simulink model "LEGO_SW"  (R2023a)
settings: Solver=VariableStepAuto  StartTime=0.0  StopTime=45  RelTol=1e-3  EnableMultiTasking=on
values from neighbouring files (symbols this model uses):
  A1 = [0,0,1,0 ... (first row only)    [run_LEGO_SW.m]
  A2 = [0,1;0,-W^2/(2*R^2)*(Kfrac+b+b_bar)/Denom]    [run_LEGO_SW.m]
  B1 = [0;0;2*(M*R*L+M*L^2+Jpsi)*Kt/Rdc/q;-2*((2*m+M)*R^2+2*J+M*R*L)*Kt/Rdc/q]    [run_LEGO_SW.m]
  B2 = [0;-W/R*Kt/Rdc/Denom]    [run_LEGO_SW.m]
  C1 = [1,0,0,0;0,0,0,1]    [run_LEGO_SW.m]
  C2 = [1,0]    [run_LEGO_SW.m]
  D1 = [0;0]    [run_LEGO_SW.m]
  D2 = 0    [run_LEGO_SW.m]
  KDtheta = -1    [run_LEGO_SW.m]
  KIpsi = -100    [run_LEGO_SW.m]
  KItheta = w_0^2*KDtheta    (= -0.8464)    [run_LEGO_SW.m]
  Kopenloop = -A2(2,2)/B2(2,1)    [run_LEGO_SW.m]
  KPphi = 6    [run_LEGO_SW.m]
  KPpsi = -10    [run_LEGO_SW.m]
  KPtheta = KDtheta * 2 * w_0 * zeta    (= -0.92)    [run_LEGO_SW.m]
  R = 0.027    [run_LEGO_SW.m]
undefined symbols (not defined in the file or in its folder): sigbuilder_block
libraries: slpidlib x2
settings Model: Creator=KostasM  LastModifiedBy=Lab5
settings SolverCC: AlgebraicLoopSolver=TrustRegion
settings DataIOCC: LimitDataPoints=on  ReturnWorkspaceOutputs=off
settings OptimizationCC: LifeSpan=inf
settings DebuggingCC: UnconnectedInputMsg=warning  UnconnectedOutputMsg=warning  UnconnectedLineMsg=warning  AllowSymbolicDim=off  SFUnexpectedBacktrackingDiag=warning  SFNoUnconditionalDefaultTransitionDiag=warning  SFExecutionAtInitializationDiag=none  ArithmeticOperatorsInVariantConditions=warning
settings ModelReferenceCC: EnableRefExpFcnMdlSchedulingChecks=on  PropagateSignalLabelsOutOfModel=off
settings SFSimCC: SimUseLocalCustomCode=off  CustomCodeUndefinedFunction=UseInterfaceOnly
settings RTWCC: RTWUseLocalCustomCode=off  DLArmComputeVersion=19.05
settings CodeAppCC: StateflowObjectComments=on
settings GRTTargetCC: TargetLangStandard=C89/C90 (ANSI)
settings ConfigComp: CovMetricSettings=dw  CovSaveCumulativeToWorkspaceVar=on  CovSaveSingleToWorkspaceVar=on  CovExternalEMLEnable=off

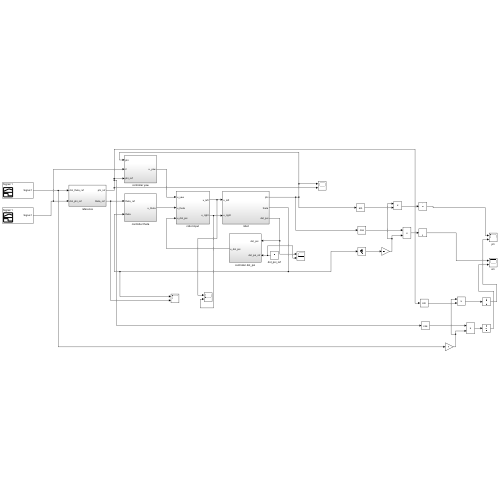
[thumbnail: Simulink's stored preview of the top-level diagram]
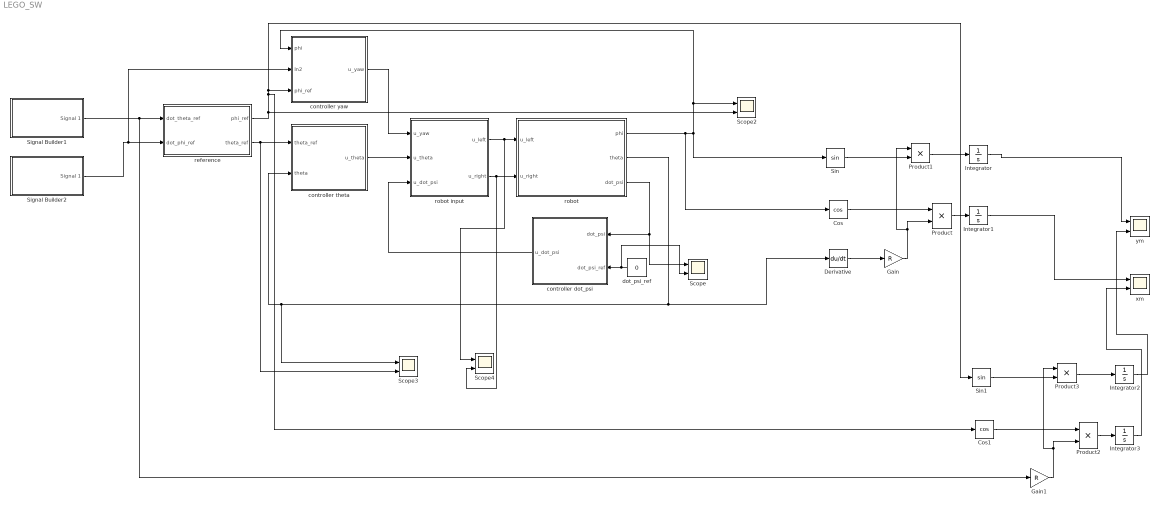
== system LEGO_SW ==
  Cos : Trigonometry  Operator=cos
  Cos1 : Trigonometry  Operator=cos
  Derivative : Derivative
  Gain : Gain  Gain=R
  Gain1 : Gain  Gain=R
  Integrator{,1..3} (4 alike) : Integrator
  Product{,1..3} (4 alike) : Product
  Scope{,2..4} (4 alike) : Scope  NumInputPorts=2
  Signal Builder1 : Subsystem  Tag=STV Subsys  LoadFcn=sigbuilder_block('load');  StartFcn=sigbuilder_block('start');  StopFcn=sigbuilder_block('stop');  ClipboardFcn=sigbuilder_block('clipboard');  mask(Sigbuilder block){tuvar=[0:10]}
      mask help: Sigbuilder GUI
      mask init:
      | if ~strcmp(get_param(bdroot(gcbh),'SimulationStatus'),'stopped') tuvar = sigbuilder_block('maskInit'); end
      settings: CopyFcn=sigbuilder_block('copy');  DeleteFcn=sigbuilder_block('delete');  ModelCloseFcn=sigbuilder_block('modelClose');  PreSaveFcn=sigbuilder_block('preSave');  PauseFcn=sigbuilder_block('pause')  ContinueFcn=sigbuilder_block('continue')  NameChangeFcn=sigbuilder_block('namechange');  OpenFcn=sigbuilder_block('open',[181.5 38.5 516 349.5 ]);  CloseFcn=sigbuilder_block('close');
      mask Display: plot(0, 0, 100, 100,[2, 2, 32, 32, 2], [68, 8, 8, 68, 68],[32, 2], [38, 38], [32, 19, 2],[53, 60, 44], [32, 17, 17, 2],[16, 16, 31, 31]);txt = getActiveGroup(gcbh);text(2, 100, txt,'verticalAlignment', 'top');
  Signal Builder2 : Subsystem  Tag=STV Subsys  LoadFcn=sigbuilder_block('load');  StartFcn=sigbuilder_block('start');  StopFcn=sigbuilder_block('stop');  ClipboardFcn=sigbuilder_block('clipboard');  mask(Sigbuilder block){tuvar=[0:10]}
      mask help: Sigbuilder GUI
      mask init:
      | if ~strcmp(get_param(bdroot(gcbh),'SimulationStatus'),'stopped') tuvar = sigbuilder_block('maskInit'); end
      settings: CopyFcn=sigbuilder_block('copy');  DeleteFcn=sigbuilder_block('delete');  ModelCloseFcn=sigbuilder_block('modelClose');  PreSaveFcn=sigbuilder_block('preSave');  PauseFcn=sigbuilder_block('pause')  ContinueFcn=sigbuilder_block('continue')  NameChangeFcn=sigbuilder_block('namechange');  OpenFcn=sigbuilder_block('open',[181.5 38.5 516 349.5 ]);  CloseFcn=sigbuilder_block('close');
      mask Display: plot(0, 0, 100, 100,[2, 2, 32, 32, 2], [68, 8, 8, 68, 68],[32, 2], [38, 38], [32, 19, 2],[53, 60, 44], [32, 17, 17, 2],[16, 16, 31, 31]);txt = getActiveGroup(gcbh);text(2, 100, txt,'verticalAlignment', 'top');
  Sin : Trigonometry
  Sin1 : Trigonometry
  controller dot_psi : Subsystem
  controller theta : Subsystem
  controller yaw : Subsystem
  dot_psi_ref : Constant  Value=0  VectorParams1D=off
  reference : Subsystem
  robot : Subsystem
  robot input : Subsystem
  xm : Scope  NumInputPorts=2
  ym : Scope  NumInputPorts=2
  wires:
  robot/3(dot_psi) -> controller dot_psi/1("dot_psi "), Scope/1
  robot input/1(u_left) -> Scope4/1, robot/1(u_left)
  robot input/2(u_right) -> Scope4/2, robot/2(u_right)
  controller theta/1(u_theta) -> robot input/2(u_theta)
  controller yaw/1(u_yaw) -> robot input/1(u_yaw)
  reference/1(phi_ref) -> Scope2/2, Cos1/1, Sin1/1, controller yaw/3(phi_ref)
  reference/2("theta_ref ") -> Scope3/2, controller theta/1(theta_ref)
  robot/2(theta) -> controller theta/2("theta "), Scope3/1, Derivative/1
  controller dot_psi/1(u_dot_psi) -> robot input/3(u_dot_psi)
  dot_psi_ref/1 -> Scope/2, controller dot_psi/2(dot_psi_ref)
  robot/1(phi) -> Cos/1, Sin/1, Scope2/1, controller yaw/1(phi)
  Signal Builder2/1(Signal 1) -> controller yaw/2(In2), reference/2("dot_phi_ref ")
  Derivative/1 -> Gain/1
  Sin/1 -> Product1/2
  Cos/1 -> Product/1
  Gain/1 -> Product1/1, Product/2
  Product1/1 -> Integrator/1
  Product/1 -> Integrator1/1
  Integrator/1 -> ym/1
  Integrator1/1 -> xm/1
  Gain1/1 -> Product3/1, Product2/2
  Signal Builder1/1(Signal 1) -> Gain1/1, reference/1("dot_theta_ref ")
  Integrator2/1 -> ym/2
  Sin1/1 -> Product3/2
  Product2/1 -> Integrator3/1
  Product3/1 -> Integrator2/1
  Integrator3/1 -> xm/2
  Cos1/1 -> Product2/1

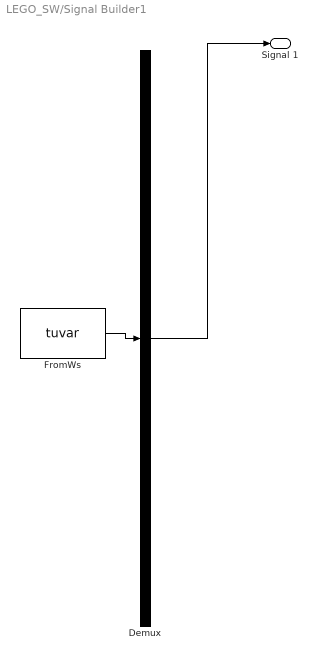
== system LEGO_SW/Signal Builder1 ==
  Demux : Demux  Tag=STV Demux  Outputs=1
      settings: DisplayOption=none
  FromWs : FromWorkspace  Tag=STV FromWs  VariableName=tuvar
      SigBuilderData=|
      | common.afterFinalStr = 'Extrapolate'
      | common.sampleTime = 0
      | dataSet.timeRange = [0 25]
      | dataSet.name = 'Signal 1'
      | sbobj.Groups.Name = 'Signal 1'
      | sbobj.Groups.Signals.Name = 'Signal 1'
      | sbobj.Groups.Signals.XData = [0 25]
      | sbobj.Groups.Signals.YData = [0 0]
      | sbobj.Groups.TimeRange = [0 25]
  Signal 1 : Outport  Tag=STV Outport
  wires:
  FromWs/1 -> Demux/1
  Demux/1 -> Signal 1/1

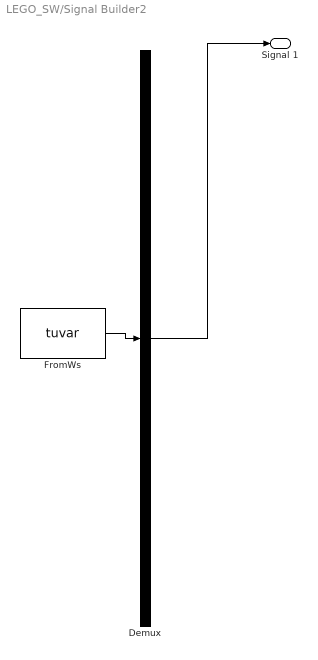
== system LEGO_SW/Signal Builder2 ==
  Demux : Demux  Tag=STV Demux  Outputs=1
      settings: DisplayOption=none
  FromWs : FromWorkspace  Tag=STV FromWs  VariableName=tuvar
      SigBuilderData=|
      | common.afterFinalStr = 'Extrapolate'
      | common.sampleTime = 0
      | dataSet.timeRange = [0 25]
      | dataSet.name = 'Signal 1'
      | sbobj.Groups.Name = 'Signal 1'
      | sbobj.Groups.Signals.Name = 'Signal 1'
      | sbobj.Groups.Signals.XData = [0 12.5 12.5 25]
      | sbobj.Groups.Signals.YData = [0 0 1 1]
      | sbobj.Groups.TimeRange = [0 25]
  Signal 1 : Outport  Tag=STV Outport
  wires:
  FromWs/1 -> Demux/1
  Demux/1 -> Signal 1/1

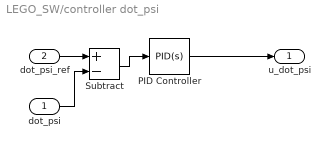
== system LEGO_SW/controller dot_psi ==
  "dot_psi " : Inport
  dot_psi_ref : Inport  Port=2
  PID Controller : slpidlib/PID Controller  Controller=PID  Form=Parallel  TimeDomain=Continuous-time  UseExternalTs=off  SampleTime=-1  IntegratorMethod=Forward Euler  FilterMethod=Forward Euler  ControllerParametersSource=internal  P=KPpsi  I=KIpsi  UseKiTs=off  D=0  N=100  UseFilter=on  TunerSelectOption=Transfer Function Based (PID Tuner App)  InitialConditionSource=internal  InitialConditionForIntegrator=0  InitialConditionForFilter=0  DifferentiatorICPrevScaledInput=0  ExternalReset=none  TrackingMode=off  Kt=1  LimitOutput=off  SatLimitsSource=internal  UpperSaturationLimit=inf  LowerSaturationLimit=-inf  LinearizeAsGain=on  AntiWindupMode=none  Kb=1  LimitIntegrator=off  UpperIntegratorSaturationLimit=inf  LowerIntegratorSaturationLimit=-inf  POutMin=[]  POutMax=[]  IOutMin=[]  IOutMax=[]  DOutMin=[]  DOutMax=[]  NOutMin=[]  NOutMax=[]  SumOutMin=[]  SumOutMax=[]  SaturationOutMin=[]  SaturationOutMax=[]  PParamMin=[]  PParamMax=[]  IParamMin=[]  IParamMax=[]  DParamMin=[]  DParamMax=[]  NParamMin=[]  NParamMax=[]  KbParamMin=[]  KbParamMax=[]  KtParamMin=[]  KtParamMax=[]  KbOutMin=[]  KbOutMax=[]  KtOutMin=[]  KtOutMax=[]  IntegratorOutMin=[]  IntegratorOutMax=[]  FilterOutMin=[]  FilterOutMax=[]  SumI1OutMin=[]  SumI1OutMax=[]  SumI2OutMin=[]  SumI2OutMax=[]  SumI3OutMin=[]  SumI3OutMax=[]  SumI4OutMin=[]  SumI4OutMax=[]  SumDOutMin=[]  SumDOutMax=[]  DifferentiatorOutMin=[]  DifferentiatorOutMax=[]  FilterDiffOutCoefMin=[]  FilterDiffOutCoefMax=[]  ReciprocalOutMin=[]  ReciprocalOutMax=[]  SumDenOutMin=[]  SumDenOutMax=[]  SumNumOutMin=[]  SumNumOutMax=[]  DivideOutMin=[]  DivideOutMax=[]  UdiffTsProdOutMin=[]  UdiffTsProdOutMax=[]  NTsProdOutMin=[]  NTsProdOutMax=[]  UintegralTsProdOutMin=[]  UintegralTsProdOutMax=[]  UngainTsProdOutMin=[]  UngainTsProdOutMax=[]  ClampingZeroOutDataTypeStr=Inherit: Inherit via back propagation  ClampingZeroOutMin=[]  ClampingZeroOutMax=[]  FilterDenConstantOutDataTypeStr=Inherit: Inherit via back propagation  FilterDenConstantOutMin=[]  FilterDenConstantOutMax=[]  PCopyOutDataTypeStr=Inherit: Inherit via back propagation  PCopyOutMin=[]  PCopyOutMax=[]  NCopyOutDataTypeStr=Inherit: Inherit via back propagation  NCopyOutMin=[]  NCopyOutMax=[]  IntegratorContinuousStateAttributes=''  IntegratorStateMustResolveToSignalObject=off  IntegratorRTWStateStorageClass=Auto  FilterContinuousStateAttributes=''  FilterStateMustResolveToSignalObject=off  FilterRTWStateStorageClass=Auto  ParallelPVariant=InternalParameters  IdealPVariant=Disabled  IVariant=InternalParameters  DVariant=InternalParameters  IntegratorVariant=Continuous  SatVariant=Disabled  AWVariant=Passthrough  PCopyVariant=Disabled  TRVariant=Disabled  FdbkBlocksVariant=Forward  IdealPFdbkVariant=Disabled  SatFdbkVariant=Disabled  DerivativeFilterVariant=ContFilter  NVariant=InternalParameters  NCopyVariant=Disabled  FilterICVariant=InternalICsFilter  IntegratorICVariant=InternalICs  ExternalResetVariant=Disabled  TRSumVariant=Passthrough  SumFdbkVariant=Disabled  SumVariant=Sum_PID  TsampFilterVariant=InternalTs  TsampNgainVariant=Passthrough  TsampIntegralVariant=Disabled_SignalSpec  ExternalSaturationOutDataTypeStr=Inherit: Same as second input
  Subtract : Sum  Inputs=+-
  u_dot_psi : Outport
  wires:
  PID Controller/1 -> u_dot_psi/1
  dot_psi_ref/1 -> Subtract/1
  Subtract/1 -> PID Controller/1
  "dot_psi "/1 -> Subtract/2

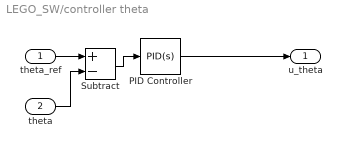
== system LEGO_SW/controller theta ==
  theta_ref : Inport
  "theta " : Inport  Port=2
  PID Controller : slpidlib/PID Controller  Controller=PID  Form=Parallel  TimeDomain=Continuous-time  UseExternalTs=off  SampleTime=-1  IntegratorMethod=Forward Euler  FilterMethod=Forward Euler  ControllerParametersSource=internal  P=KPtheta  I=KItheta  UseKiTs=off  D=KDtheta  N=100  UseFilter=on  TunerSelectOption=Transfer Function Based (PID Tuner App)  InitialConditionSource=internal  InitialConditionForIntegrator=0  InitialConditionForFilter=0  DifferentiatorICPrevScaledInput=0  ExternalReset=none  TrackingMode=off  Kt=1  LimitOutput=off  SatLimitsSource=internal  UpperSaturationLimit=inf  LowerSaturationLimit=-inf  LinearizeAsGain=on  AntiWindupMode=none  Kb=1  LimitIntegrator=off  UpperIntegratorSaturationLimit=inf  LowerIntegratorSaturationLimit=-inf  POutMin=[]  POutMax=[]  IOutMin=[]  IOutMax=[]  DOutMin=[]  DOutMax=[]  NOutMin=[]  NOutMax=[]  SumOutMin=[]  SumOutMax=[]  SaturationOutMin=[]  SaturationOutMax=[]  PParamMin=[]  PParamMax=[]  IParamMin=[]  IParamMax=[]  DParamMin=[]  DParamMax=[]  NParamMin=[]  NParamMax=[]  KbParamMin=[]  KbParamMax=[]  KtParamMin=[]  KtParamMax=[]  KbOutMin=[]  KbOutMax=[]  KtOutMin=[]  KtOutMax=[]  IntegratorOutMin=[]  IntegratorOutMax=[]  FilterOutMin=[]  FilterOutMax=[]  SumI1OutMin=[]  SumI1OutMax=[]  SumI2OutMin=[]  SumI2OutMax=[]  SumI3OutMin=[]  SumI3OutMax=[]  SumI4OutMin=[]  SumI4OutMax=[]  SumDOutMin=[]  SumDOutMax=[]  DifferentiatorOutMin=[]  DifferentiatorOutMax=[]  FilterDiffOutCoefMin=[]  FilterDiffOutCoefMax=[]  ReciprocalOutMin=[]  ReciprocalOutMax=[]  SumDenOutMin=[]  SumDenOutMax=[]  SumNumOutMin=[]  SumNumOutMax=[]  DivideOutMin=[]  DivideOutMax=[]  UdiffTsProdOutMin=[]  UdiffTsProdOutMax=[]  NTsProdOutMin=[]  NTsProdOutMax=[]  UintegralTsProdOutMin=[]  UintegralTsProdOutMax=[]  UngainTsProdOutMin=[]  UngainTsProdOutMax=[]  ClampingZeroOutDataTypeStr=Inherit: Inherit via back propagation  ClampingZeroOutMin=[]  ClampingZeroOutMax=[]  FilterDenConstantOutDataTypeStr=Inherit: Inherit via back propagation  FilterDenConstantOutMin=[]  FilterDenConstantOutMax=[]  PCopyOutDataTypeStr=Inherit: Inherit via back propagation  PCopyOutMin=[]  PCopyOutMax=[]  NCopyOutDataTypeStr=Inherit: Inherit via back propagation  NCopyOutMin=[]  NCopyOutMax=[]  IntegratorContinuousStateAttributes=''  IntegratorStateMustResolveToSignalObject=off  IntegratorRTWStateStorageClass=Auto  FilterContinuousStateAttributes=''  FilterStateMustResolveToSignalObject=off  FilterRTWStateStorageClass=Auto  ParallelPVariant=InternalParameters  IdealPVariant=Disabled  IVariant=InternalParameters  DVariant=InternalParameters  IntegratorVariant=Continuous  SatVariant=Disabled  AWVariant=Passthrough  PCopyVariant=Disabled  TRVariant=Disabled  FdbkBlocksVariant=Forward  IdealPFdbkVariant=Disabled  SatFdbkVariant=Disabled  DerivativeFilterVariant=ContFilter  NVariant=InternalParameters  NCopyVariant=Disabled  FilterICVariant=InternalICsFilter  IntegratorICVariant=InternalICs  ExternalResetVariant=Disabled  TRSumVariant=Passthrough  SumFdbkVariant=Disabled  SumVariant=Sum_PID  TsampFilterVariant=InternalTs  TsampNgainVariant=Passthrough  TsampIntegralVariant=Disabled_SignalSpec  ExternalSaturationOutDataTypeStr=Inherit: Same as second input
  Subtract : Sum  Inputs=+-
  u_theta : Outport
  wires:
  theta_ref/1 -> Subtract/1
  "theta "/1 -> Subtract/2
  Subtract/1 -> PID Controller/1
  PID Controller/1 -> u_theta/1

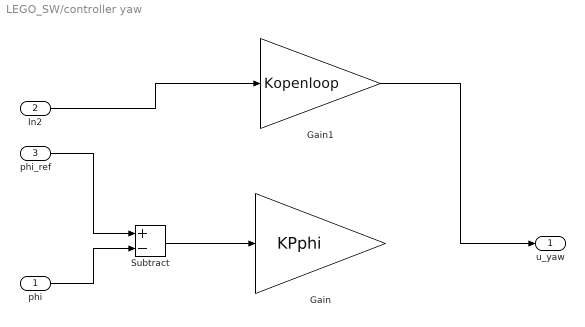
== system LEGO_SW/controller yaw ==
  phi : Inport
  In2 : Inport  Port=2
  phi_ref : Inport  Port=3
  Gain : Gain  Gain=KPphi
  Gain1 : Gain  Gain=Kopenloop
  Subtract : Sum  Inputs=+-
  u_yaw : Outport
  wires:
  Subtract/1 -> Gain/1
  phi_ref/1 -> Subtract/1
  phi/1 -> Subtract/2
  In2/1 -> Gain1/1
  Gain1/1 -> u_yaw/1

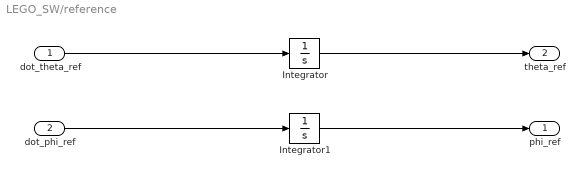
== system LEGO_SW/reference ==
  "dot_theta_ref " : Inport
  "dot_phi_ref " : Inport  Port=2
  Integrator : Integrator
  Integrator1 : Integrator
  phi_ref : Outport
  "theta_ref " : Outport  Port=2
  wires:
  "dot_theta_ref "/1 -> Integrator/1
  Integrator/1 -> "theta_ref "/1
  "dot_phi_ref "/1 -> Integrator1/1
  Integrator1/1 -> phi_ref/1

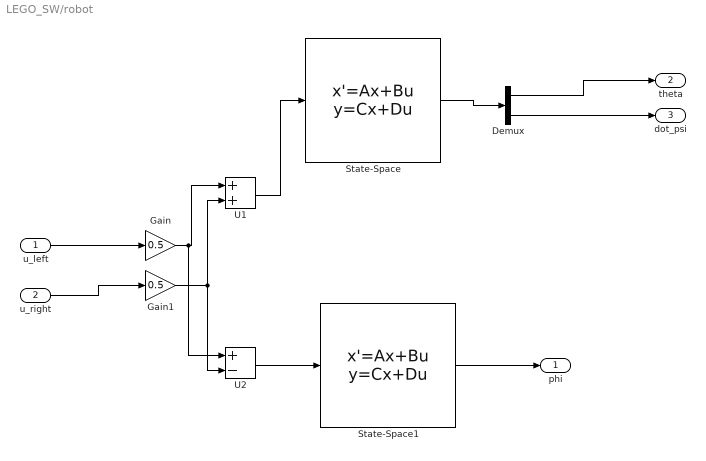
== system LEGO_SW/robot ==
  u_left : Inport
  u_right : Inport  Port=2
  Demux : Demux  Outputs=2
  Gain : Gain  Gain=0.5
  Gain1 : Gain  Gain=0.5
  State-Space : StateSpace  A=A1  B=B1  C=C1  D=D1  InitialCondition=0
  State-Space1 : StateSpace  A=A2  B=B2  C=C2  D=D2  InitialCondition=0
  U1 : Sum
  U2 : Sum  Inputs=+-
  phi : Outport
  theta : Outport  Port=2
  dot_psi : Outport  Port=3
  wires:
  u_left/1 -> Gain/1
  u_right/1 -> Gain1/1
  Gain/1 -> U2/1, U1/1
  Gain1/1 -> U2/2, U1/2
  U1/1 -> State-Space/1
  State-Space/1 -> Demux/1
  Demux/1 -> theta/1
  Demux/2 -> dot_psi/1
  U2/1 -> State-Space1/1
  State-Space1/1 -> phi/1

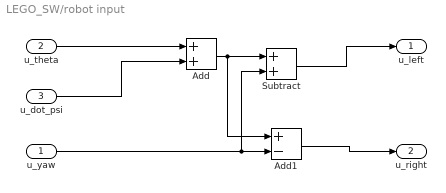
== system LEGO_SW/robot input ==
  u_yaw : Inport
  u_theta : Inport  Port=2
  u_dot_psi : Inport  Port=3
  Add : Sum
  Add1 : Sum  Inputs=+-
  Subtract : Sum
  u_left : Outport
  u_right : Outport  Port=2
  wires:
  u_theta/1 -> Add/1
  u_dot_psi/1 -> Add/2
  u_yaw/1 -> Add1/2, Subtract/2
  Add/1 -> Add1/1, Subtract/1
  Subtract/1 -> u_left/1
  Add1/1 -> u_right/1
